simulink model "attitude_estimation_AS_V4"  (Simulink 8.9)
settings: Solver=ode45  StartTime=0.0  StopTime=400  FixedStep=T  RelTol=1e-9  EnableMultiTasking=on
values from neighbouring files (symbols this model uses):
  ARW = ARWSigma*(pi/180)/sqrt(3600)    [graficosD7.m]    (also in iattitude_estimation.m = 2.9e-06; iattitude_estimation_AS.m)
  best0 = 0    [iattitude_estimation.m]    (also in iattitude_estimation_AS.m)
  bias_cte = 4.848e-6*bias_cte    [iattitude_estimation.m]    (also in iattitude_estimation_AS.m = bias_cte*(pi/(180*3600)))
  BISigma = 0    [iattitude_estimation_AS.m]
  Misalig = [ ... (first row only)    [iattitude_estimation.m]    (also in iattitude_estimation_AS.m)
  Pest0 = zeros(6,6)    [iattitude_estimation.m]    (also in iattitude_estimation_AS.m)
  Q = 1*C_bl_GYRO_aux*Q_coefs*(C_bl_GYRO_aux')    [iattitude_estimation_AS.m]
  qest0 = qest0/sqrt(qest0'*qest0)    [iattitude_estimation.m]    (also in iattitude_estimation_AS.m)
  qreal0 = qreal0/sqrt(qreal0'*qreal0)    [iattitude_estimation.m]    (also in iattitude_estimation_AS.m)
  R = 1*(1/4)*C_bl_STR*(eye(3)*(sss^2))*(C_bl_STR')    [iattitude_estimation_AS.m]
  RRW = 8e-8*RRW    (= 0)    [iattitude_estimation.m]    (also in iattitude_estimation_AS.m)
  seta1filt = 1*ARW    (= 2.9e-06)    [iattitude_estimation.m]    (also in iattitude_estimation_AS.m = 1*ARW)
  seta2filt = 1*1e-7    (= 1e-07)    [iattitude_estimation.m]    (also in iattitude_estimation_AS.m)
  So = So/(2*3.1416)    (= 185311.942959)    [iattitude_estimation.m]    (also in iattitude_estimation_AS.m = 185312.376299)
  sstar = [sss; sss; sss]    [iattitude_estimation.m]    (also in iattitude_estimation_AS.m)
  sstarfilt = 1*sstar    [iattitude_estimation.m]    (also in iattitude_estimation_AS.m)
  T = 1    [iattitude_estimation.m]    (also in iattitude_estimation_AS.m)
  Tgyro = T/1    (= 1)    [iattitude_estimation.m]    (also in iattitude_estimation_AS.m = 0.1)
libraries: dspsrcs4 x1, simulink x1
settings Model: SuppressorTable=22 serialization::archive 11 0 6 0 0 0 11 0  Creator=INVAP  LastModifiedBy=root
settings DataIOCC: SignalLoggingName=sigsOut
settings DebuggingCC: SaveWithParameterizedLinksMsg=none  SignalResolutionControl=TryResolveAllWithWarning  MultiTaskDSMMsg=warning  MultiTaskCondExecSysMsg=none  FcnCallInpInsideContextMsg=error  StateNameClashWarn=none
settings HardwareCC: TargetUnknown=on
settings ConfigComp: CovSFcnEnable=off

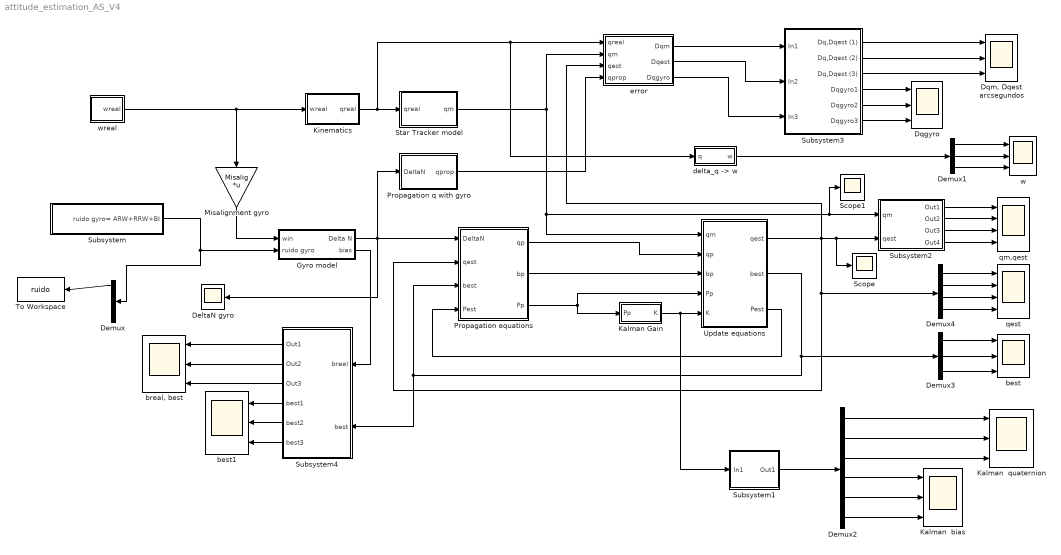
== system attitude_estimation_AS_V4 ==
  DeltaN gyro : Scope
  Demux : Demux  Outputs=3
  Demux1 : Demux  Outputs=3
  Demux2 : Demux  Outputs=6
  Demux3 : Demux  Outputs=3
  Demux4 : Demux
  Dqgyro : Scope  NumInputPorts=3
  "Dqm, Dqest arcsegundos" : Scope  NumInputPorts=3
  Gyro model : Subsystem
  Kalman Gain : Subsystem
  Kalman  bias : Scope  NumInputPorts=3
  Kalman  quaternion : Scope  NumInputPorts=3
  Kinematics : Subsystem
  Misalignment gyro : Gain  Gain=Misalig  Multiplication=Matrix(K*u) (u vector)  SaturateOnIntegerOverflow=on  OutDataTypeStr=Inherit: Same as input  ParamDataTypeStr=Inherit: Same as input
  Propagation equations : Subsystem
  Propagation q with gyro : Subsystem
  Scope : Scope
  Scope1 : Scope
  Star Tracker model : Subsystem
  Subsystem : Subsystem
  Subsystem1 : Subsystem
  Subsystem2 : Subsystem
  Subsystem3 : Subsystem
  Subsystem4 : Subsystem
  To Workspace : ToWorkspace  VariableName=ruido  SaveFormat=Timeseries  SampleTime=-1
  Update equations : Subsystem
  best : Scope  NumInputPorts=3
  best1 : Scope  NumInputPorts=3
  "breal, best" : Scope  NumInputPorts=3
  "delta_q -> w" : Subsystem
  error : Subsystem
  qest : Scope  NumInputPorts=4
  qm,qest : Scope  NumInputPorts=4
  w : Scope  NumInputPorts=3
  wreal : Subsystem
  wires:
  Kinematics/1(qreal) -> Star Tracker model/1(qreal), "delta_q -> w"/1(q), error/1(qreal)
  wreal/1(wreal) -> Kinematics/1(wreal), Misalignment gyro/1
  Star Tracker model/1(qm) -> error/2(qm), Update equations/1(qm), Scope1/1, Subsystem2/1(qm)
  Propagation equations/1(qp) -> Update equations/2(qp)
  Kalman Gain/1(K) -> Update equations/5(K), Subsystem1/1(In1)
  Update equations/3(Pest) -> Propagation equations/4(Pest)
  Update equations/1(qest) -> error/3(qest), Scope/1, Subsystem2/2(qest), Propagation equations/2(qest), Demux4/1
  Gyro model/1(Delta N) -> Propagation equations/1(DeltaN), Propagation q with gyro/1(DeltaN), DeltaN gyro/1
  Propagation q with gyro/1(qprop) -> error/4(qprop)
  Propagation equations/2(bp) -> Update equations/3(bp)
  Propagation equations/3(Pp) -> Update equations/4(Pp), Kalman Gain/1(Pp)
  Misalignment gyro/1 -> Gyro model/1(win)
  Update equations/2(best) -> Subsystem4/2(best), Propagation equations/3(best), Demux3/1
  Subsystem/1(ruido gyro= ARW+RRW+BI) -> Gyro model/2(ruido gyro), Demux/1
  Demux2/1 -> Kalman  quaternion/1
  Demux2/2 -> Kalman  quaternion/2
  Demux2/3 -> Kalman  quaternion/3
  Demux2/5 -> Kalman  bias/2
  Demux2/4 -> Kalman  bias/1
  Demux3/2 -> best/2
  Demux4/1 -> qest/1
  Demux4/2 -> qest/2
  Demux4/3 -> qest/3
  Subsystem1/1(Out1) -> Demux2/1
  Demux4/4 -> qest/4
  Subsystem2/1(Out1) -> qm,qest/1
  Subsystem2/2(Out2) -> qm,qest/2
  Subsystem2/3(Out3) -> qm,qest/3
  Subsystem2/4(Out4) -> qm,qest/4
  error/1(Dqm) -> Subsystem3/1(In1)
  error/2(Dqest) -> Subsystem3/2(In2)
  error/3(Dqgyro) -> Subsystem3/3(In3)
  Subsystem3/1(Dq,Dqest (1)) -> "Dqm, Dqest arcsegundos"/1
  Subsystem3/2(Dq,Dqest (2)) -> "Dqm, Dqest arcsegundos"/2
  Subsystem3/3(Dq,Dqest (3)) -> "Dqm, Dqest arcsegundos"/3
  Gyro model/2(bias) -> Subsystem4/1(breal)
  Subsystem3/4(Dqgyro1) -> Dqgyro/1
  Subsystem3/5(Dqgyro2) -> Dqgyro/2
  Subsystem3/6(Dqgyro3) -> Dqgyro/3
  "delta_q -> w"/1(w) -> Demux1/1
  Demux1/2 -> w/2
  Demux1/3 -> w/3
  Demux1/1 -> w/1
  Demux3/1 -> best/1
  Demux3/3 -> best/3
  Demux2/6 -> Kalman  bias/3
  Subsystem4/5(best2) -> best1/2
  Subsystem4/4(best1) -> best1/1
  Subsystem4/6(best3) -> best1/3
  Subsystem4/1(Out1) -> "breal, best"/1
  Subsystem4/2(Out2) -> "breal, best"/2
  Subsystem4/3(Out3) -> "breal, best"/3
  Demux/1 -> To Workspace/1

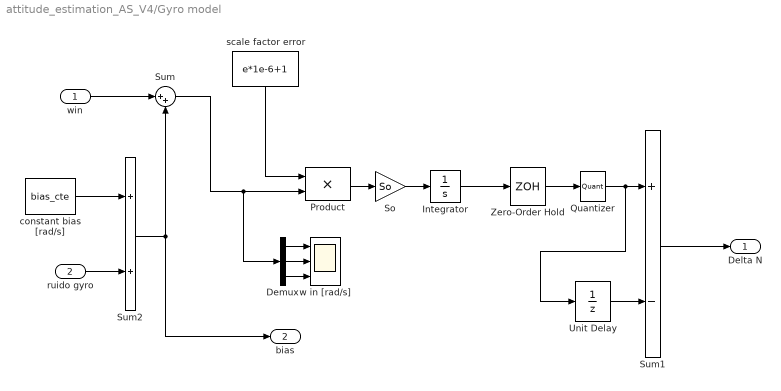
== system attitude_estimation_AS_V4/Gyro model ==
  win : Inport
  ruido gyro : Inport  Port=2
  Demux : Demux  Outputs=3
  Integrator : Integrator
  Product : Product  SaturateOnIntegerOverflow=on  OutDataTypeStr=Inherit: Same as first input
  Quantizer : Quantizer  QuantizationInterval=1
  So : Gain  Gain=So  SaturateOnIntegerOverflow=on  OutDataTypeStr=Inherit: Same as input  ParamDataTypeStr=Inherit: Same as input
  Sum : Sum  Inputs=|++  SaturateOnIntegerOverflow=on
  Sum1 : Sum  Inputs=+-  SaturateOnIntegerOverflow=on
  Sum2 : Sum  SaturateOnIntegerOverflow=on
  Unit Delay : UnitDelay  SampleTime=Tgyro
  Zero-Order Hold : ZeroOrderHold  SampleTime=Tgyro
  constant bias [rad/s] : Constant  Value=bias_cte
  scale factor error : Constant  Value=e*1e-6+1
  w in [rad/s] : Scope  NumInputPorts=3
  Delta N : Outport
  bias : Outport  Port=2
  wires:
  So/1 -> Integrator/1
  Product/1 -> So/1
  scale factor error/1 -> Product/1
  Zero-Order Hold/1 -> Quantizer/1
  Unit Delay/1 -> Sum1/2
  Integrator/1 -> Zero-Order Hold/1
  Sum1/1 -> Delta N/1
  Quantizer/1 -> Sum1/1, Unit Delay/1
  Sum2/1 -> Sum/2, bias/1
  ruido gyro/1 -> Sum2/2
  win/1 -> Sum/1
  Demux/1 -> w in [rad/s]/1
  Demux/2 -> w in [rad/s]/2
  Demux/3 -> w in [rad/s]/3
  Sum/1 -> Demux/1, Product/2
  constant bias [rad/s]/1 -> Sum2/1

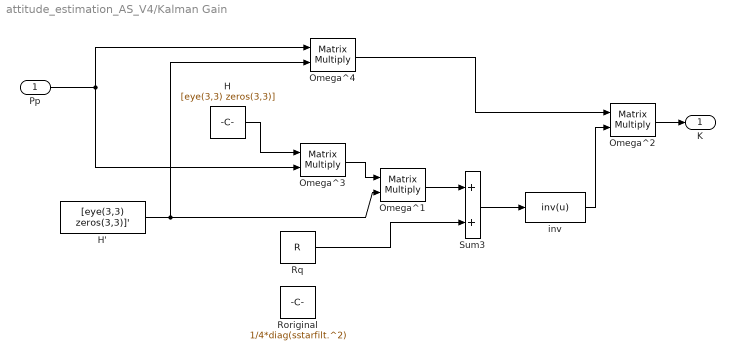
== system attitude_estimation_AS_V4/Kalman Gain ==
  Pp : Inport
  H : Constant  Value=[eye(3,3) zeros(3,3)]  VectorParams1D=off
  H' : Constant  Value=[eye(3,3) zeros(3,3)]'  VectorParams1D=off
  Omega^{1..4} (4 alike) : Product  Multiplication=Matrix(*)  SaturateOnIntegerOverflow=on  OutDataTypeStr=Inherit: Same as first input
  Roriginal : Constant  Value=1/4*diag(sstarfilt.^2)  VectorParams1D=off
  Rq : Constant  Value=R  VectorParams1D=off
  Sum3 : Sum  SaturateOnIntegerOverflow=on
  inv : MATLABFcn  MATLABFcn=inv(u)  Output1D=off
  K : Outport
  wires:
  H/1 -> Omega^3/1
  Pp/1 -> Omega^3/2, Omega^4/1
  Omega^3/1 -> Omega^1/1
  H'/1 -> Omega^1/2, Omega^4/2
  Omega^1/1 -> Sum3/1
  Omega^2/1 -> K/1
  Omega^4/1 -> Omega^2/1
  Sum3/1 -> inv/1
  inv/1 -> Omega^2/2
  Rq/1 -> Sum3/2

== system attitude_estimation_AS_V4/Kinematics ==
  wreal : Inport
  Integrator : Integrator  InitialCondition=qreal0
  MATLAB Fcn : MATLABFcn  MATLABFcn=1/2*[0 u(3) -u(2) u(1); -u(3) 0 u(1) u(2); u(2) -u(1) 0 u(3); -u(1) -u(2) -u(3) 0]  Output1D=off
  Product : Product  Multiplication=Matrix(*)  SaturateOnIntegerOverflow=on  OutDataTypeStr=Inherit: Same as first input
  qreal : Outport
  wires:
  wreal/1 -> MATLAB Fcn/1
  MATLAB Fcn/1 -> Product/1
  Product/1 -> Integrator/1
  Integrator/1 -> Product/2, qreal/1

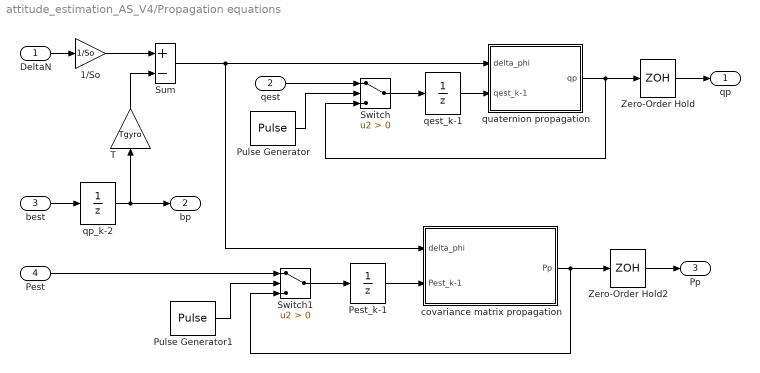
== system attitude_estimation_AS_V4/Propagation equations ==
  DeltaN : Inport
  qest : Inport  Port=2
  best : Inport  Port=3
  Pest : Inport  Port=4
  1/So : Gain  Gain=1/So  SaturateOnIntegerOverflow=on  OutDataTypeStr=Inherit: Same as input  ParamDataTypeStr=Inherit: Same as input
  Pest_k-1 : UnitDelay  InitialCondition=Pest0  SampleTime=Tgyro
  Pulse Generator : DiscretePulseGenerator  Period=T/Tgyro  SampleTime=Tgyro
  Pulse Generator1 : DiscretePulseGenerator  Period=T/Tgyro  SampleTime=Tgyro
  Sum : Sum  Inputs=+-  SaturateOnIntegerOverflow=on
  Switch : Switch  Criteria=u2 > Threshold  SaturateOnIntegerOverflow=on
  Switch1 : Switch  Criteria=u2 > Threshold  SaturateOnIntegerOverflow=on
  T : Gain  Gain=Tgyro  SaturateOnIntegerOverflow=on  OutDataTypeStr=Inherit: Same as input  ParamDataTypeStr=Inherit: Same as input
  Zero-Order Hold : ZeroOrderHold  SampleTime=T
  Zero-Order Hold2 : ZeroOrderHold  SampleTime=T
  covariance matrix propagation : Subsystem
  qest_k-1 : UnitDelay  InitialCondition=qest0  SampleTime=Tgyro
  qp_k-2 : UnitDelay  InitialCondition=best0  SampleTime=T
  quaternion propagation : Subsystem
  qp : Outport
  bp : Outport  Port=2
  Pp : Outport  Port=3
  wires:
  DeltaN/1 -> 1/So/1
  Sum/1 -> quaternion propagation/1(delta_phi), covariance matrix propagation/1(delta_phi)
  quaternion propagation/1(qp) -> Zero-Order Hold/1, Switch/3
  T/1 -> Sum/2
  1/So/1 -> Sum/1
  covariance matrix propagation/1(Pp) -> Zero-Order Hold2/1, Switch1/3
  Zero-Order Hold/1 -> qp/1
  qest/1 -> Switch/1
  Pulse Generator/1 -> Switch/2
  qest_k-1/1 -> quaternion propagation/2(qest_k-1)
  Switch/1 -> qest_k-1/1
  Pest_k-1/1 -> covariance matrix propagation/2(Pest_k-1)
  best/1 -> qp_k-2/1
  qp_k-2/1 -> bp/1, T/1
  Zero-Order Hold2/1 -> Pp/1
  Switch1/1 -> Pest_k-1/1
  Pest/1 -> Switch1/1
  Pulse Generator1/1 -> Switch1/2

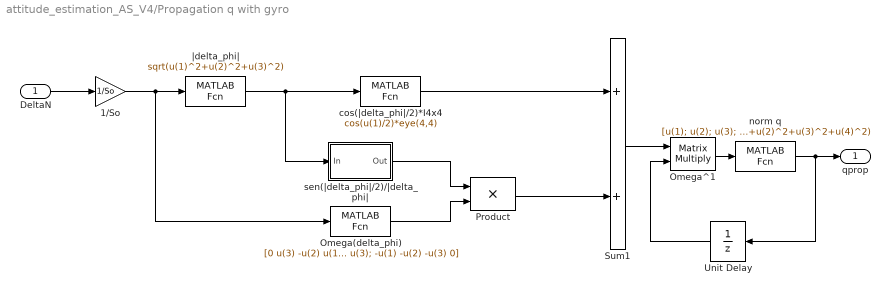
== system attitude_estimation_AS_V4/Propagation q with gyro ==
  DeltaN : Inport
  1/So : Gain  Gain=1/So  SaturateOnIntegerOverflow=on  OutDataTypeStr=Inherit: Same as input  ParamDataTypeStr=Inherit: Same as input
  Omega(delta_phi) : MATLABFcn  MATLABFcn=[0 u(3) -u(2) u(1); -u(3) 0 u(1) u(2); u(2) -u(1) 0 u(3); -u(1) -u(2) -u(3) 0]  Output1D=off
  Omega^1 : Product  Multiplication=Matrix(*)  SaturateOnIntegerOverflow=on  OutDataTypeStr=Inherit: Same as first input
  Product : Product  SaturateOnIntegerOverflow=on  OutDataTypeStr=Inherit: Same as first input
  Sum1 : Sum  SaturateOnIntegerOverflow=on
  Unit Delay : UnitDelay  InitialCondition=qreal0  SampleTime=Tgyro
  cos(|delta_phi|/2)*I4x4 : MATLABFcn  MATLABFcn=cos(u(1)/2)*eye(4,4)  Output1D=off
  norm q : MATLABFcn  MATLABFcn=[u(1); u(2); u(3); u(4)]/sqrt(u(1)^2+u(2)^2+u(3)^2+u(4)^2)  Output1D=off
  sen(|delta_phi|/2)/|delta_phi| : Subsystem
  |delta_phi| : MATLABFcn  MATLABFcn=sqrt(u(1)^2+u(2)^2+u(3)^2)  Output1D=off
  qprop : Outport
  wires:
  DeltaN/1 -> 1/So/1
  Omega^1/1 -> norm q/1
  norm q/1 -> qprop/1, Unit Delay/1
  Sum1/1 -> Omega^1/1
  Unit Delay/1 -> Omega^1/2
  |delta_phi|/1 -> cos(|delta_phi|/2)*I4x4/1, sen(|delta_phi|/2)/|delta_phi|/1(In)
  1/So/1 -> |delta_phi|/1, Omega(delta_phi)/1
  cos(|delta_phi|/2)*I4x4/1 -> Sum1/1
  Product/1 -> Sum1/2
  sen(|delta_phi|/2)/|delta_phi|/1(Out) -> Product/1
  Omega(delta_phi)/1 -> Product/2

== system attitude_estimation_AS_V4/Star Tracker model ==
  qreal : Inport
  Product : Product  Multiplication=Matrix(*)  SaturateOnIntegerOverflow=on  OutDataTypeStr=Inherit: Same as first input
  Qprim : MATLABFcn  MATLABFcn=[u(4) u(3) -u(2) u(1); -u(3) u(4) u(1) u(2); u(2) -u(1) u(4) u(3); -u(1) -u(2) -u(3) u(4)]  Output1D=off
  Zero-Order Hold : ZeroOrderHold  SampleTime=T
  "noise pitch, yaw, roll" : RandomNumber  Variance=sstar.^2  Seed=rand(3,1)*100  SampleTime=T  VectorParams1D=off
  noise_q : MATLABFcn  MATLABFcn=[1/2*u(1); 1/2*u(2); 1/2*u(3); 1]  Output1D=off
  normalition qm : MATLABFcn  MATLABFcn=[u(1); u(2); u(3); u(4)]/sqrt(u(1)^2+u(2)^2+u(3)^2+u(4)^2)  Output1D=off
  qm : Outport
  wires:
  "noise pitch, yaw, roll"/1 -> noise_q/1
  noise_q/1 -> Qprim/1
  Qprim/1 -> Product/1
  qreal/1 -> Zero-Order Hold/1
  Product/1 -> normalition qm/1
  normalition qm/1 -> qm/1
  Zero-Order Hold/1 -> Product/2

== system attitude_estimation_AS_V4/Subsystem ==
  Colored Noise : dspsrcs4/Colored Noise  Color=pink  InverseFrequencyPower=1  NumChannels=1  OutputDataType=double  SamplesPerFrame=1  SampleTime=Tgyro  RandomStream=mt19937ar with seed  Seed=67  SimulateUsing=Interpreted execution
      settings: SourceProductName=DSP System Toolbox  SourceProductBaseCode=DS
  Gain1 : Gain  Gain=ARW
  Gain2 : Gain  Gain=RRW
  Gain3 : Gain  Gain=BISigma/3600
  Integrator : Integrator
  Interpreted MATLAB Function : MATLABFcn  MATLABFcn=[u;u;u]  Output1D=off
  Random Number : RandomNumber  SampleTime=Tgyro
  Sum : Sum  Inputs=+++
  ruido gyro= ARW+RRW+BI : Outport
  wires:
  Random Number/1 -> Gain1/1, Gain2/1
  Sum/1 -> Interpreted MATLAB Function/1
  Gain1/1 -> Sum/1  "Angle random walk"
  Gain2/1 -> Integrator/1
  Interpreted MATLAB Function/1 -> ruido gyro= ARW+RRW+BI/1
  Colored Noise/1 -> Gain3/1
  Integrator/1 -> Sum/2  "Rate random walk"
  Gain3/1 -> Sum/3  "Bias instability"

== system attitude_estimation_AS_V4/Subsystem1 ==
  In1 : Inport
  Interpreted MATLAB Function : MATLABFcn  MATLABFcn=[u(1,1);u(2,2);u(3,3);u(4,1);u(5,2);u(6,3)]  Output1D=off
  Out1 : Outport
  wires:
  In1/1 -> Interpreted MATLAB Function/1
  Interpreted MATLAB Function/1 -> Out1/1

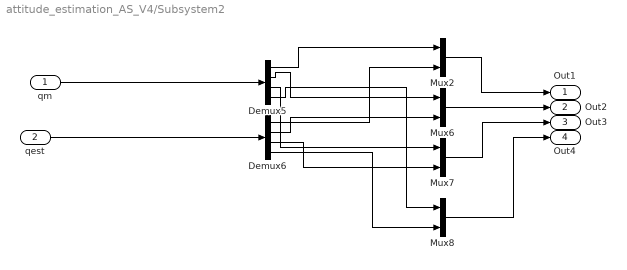
== system attitude_estimation_AS_V4/Subsystem2 ==
  qm : Inport
  qest : Inport  Port=2
  Demux5 : Demux
  Demux6 : Demux
  Mux{2,6..8} (4 alike) : Mux  Inputs=2
  Out1 : Outport
  Out2 : Outport  Port=2
  Out3 : Outport  Port=3
  Out4 : Outport  Port=4
  wires:
  qest/1 -> Demux6/1
  Demux6/3 -> Mux7/2
  Mux8/1 -> Out4/1
  Demux5/4 -> Mux8/1
  Demux5/3 -> Mux7/1
  Mux7/1 -> Out3/1
  Demux6/2 -> Mux6/2
  Demux6/4 -> Mux8/2
  qm/1 -> Demux5/1
  Demux5/1 -> Mux2/1
  Demux6/1 -> Mux2/2
  Demux5/2 -> Mux6/1
  Mux2/1 -> Out1/1
  Mux6/1 -> Out2/1

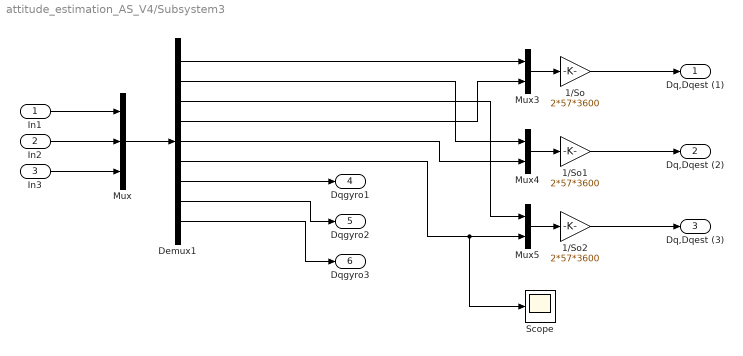
== system attitude_estimation_AS_V4/Subsystem3 ==
  In1 : Inport
  In2 : Inport  Port=2
  In3 : Inport  Port=3
  1/So : Gain  Gain=2*57*3600  SaturateOnIntegerOverflow=on  OutDataTypeStr=Inherit: Same as input  ParamDataTypeStr=Inherit: Same as input
  1/So1 : Gain  Gain=2*57*3600  SaturateOnIntegerOverflow=on  OutDataTypeStr=Inherit: Same as input  ParamDataTypeStr=Inherit: Same as input
  1/So2 : Gain  Gain=2*57*3600  SaturateOnIntegerOverflow=on  OutDataTypeStr=Inherit: Same as input  ParamDataTypeStr=Inherit: Same as input
  Demux1 : Demux  Outputs=9
  Mux : Mux  Inputs=3
  Mux3 : Mux  Inputs=2
  Mux4 : Mux  Inputs=2
  Mux5 : Mux  Inputs=2
  Scope : Scope
  Dq,Dqest (1) : Outport
  Dq,Dqest (2) : Outport  Port=2
  Dq,Dqest (3) : Outport  Port=3
  Dqgyro1 : Outport  Port=4
  Dqgyro2 : Outport  Port=5
  Dqgyro3 : Outport  Port=6
  wires:
  Demux1/8 -> Dqgyro2/1
  Demux1/2 -> Mux4/1
  1/So2/1 -> Dq,Dqest (3)/1
  Demux1/5 -> Mux4/2
  1/So1/1 -> Dq,Dqest (2)/1
  Demux1/3 -> Mux5/1
  Demux1/6 -> Scope/1, Mux5/2
  Mux5/1 -> 1/So2/1
  Demux1/4 -> Mux3/2
  Demux1/1 -> Mux3/1
  Demux1/7 -> Dqgyro1/1
  In3/1 -> Mux/3
  In2/1 -> Mux/2
  Mux/1 -> Demux1/1
  In1/1 -> Mux/1
  1/So/1 -> Dq,Dqest (1)/1
  Demux1/9 -> Dqgyro3/1
  Mux4/1 -> 1/So1/1
  Mux3/1 -> 1/So/1

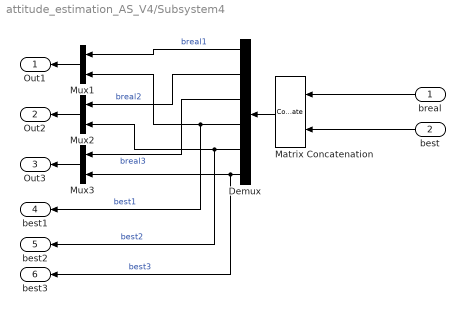
== system attitude_estimation_AS_V4/Subsystem4 ==
  breal : Inport
  best : Inport  Port=2
  Demux : Demux  Outputs=6
  Matrix Concatenation : Concatenate  Mode=Multidimensional array
  Mux1 : Mux  Inputs=2
  Mux2 : Mux  Inputs=2
  Mux3 : Mux  Inputs=2
  Out1 : Outport
  Out2 : Outport  Port=2
  Out3 : Outport  Port=3
  best1 : Outport  Port=4
  best2 : Outport  Port=5
  best3 : Outport  Port=6
  wires:
  Demux/6 -> best3/1, Mux3/2  "best3"
  Matrix Concatenation/1 -> Demux/1
  Demux/5 -> best2/1, Mux2/2  "best2"
  Mux3/1 -> Out3/1
  Mux2/1 -> Out2/1
  best/1 -> Matrix Concatenation/2
  Mux1/1 -> Out1/1
  Demux/2 -> Mux2/1  "breal2"
  Demux/4 -> best1/1, Mux1/2  "best1"
  Demux/1 -> Mux1/1  "breal1"
  breal/1 -> Matrix Concatenation/1
  Demux/3 -> Mux3/1  "breal3"

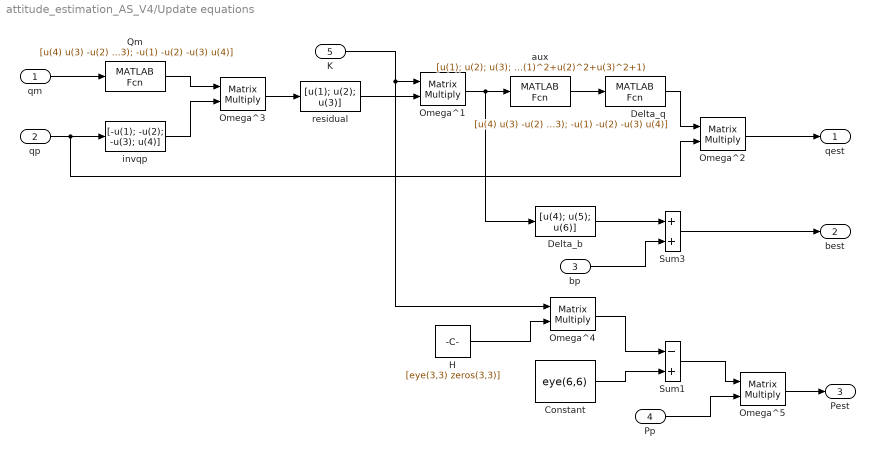
== system attitude_estimation_AS_V4/Update equations ==
  qm : Inport
  qp : Inport  Port=2
  bp : Inport  Port=3
  Pp : Inport  Port=4
  K : Inport  Port=5
  Constant : Constant  Value=eye(6,6)  VectorParams1D=off
  Delta_b : MATLABFcn  MATLABFcn=[u(4); u(5); u(6)]  Output1D=off
  Delta_q : MATLABFcn  MATLABFcn=[u(4) u(3) -u(2) u(1); -u(3) u(4) u(1) u(2); u(2) -u(1) u(4) u(3); -u(1) -u(2) -u(3) u(4)]  Output1D=off
  H : Constant  Value=[eye(3,3) zeros(3,3)]  VectorParams1D=off
  Omega^{1..5} (5 alike) : Product  Multiplication=Matrix(*)  SaturateOnIntegerOverflow=on  OutDataTypeStr=Inherit: Same as first input
  Qm : MATLABFcn  MATLABFcn=[u(4) u(3) -u(2) u(1); -u(3) u(4) u(1) u(2); u(2) -u(1) u(4) u(3); -u(1) -u(2) -u(3) u(4)]  Output1D=off
  Sum1 : Sum  Inputs=-+  SaturateOnIntegerOverflow=on
  Sum3 : Sum  SaturateOnIntegerOverflow=on
  aux : MATLABFcn  MATLABFcn=[u(1); u(2); u(3); 1]*sqrt(u(1)^2+u(2)^2+u(3)^2+1)  Output1D=off
  invqp : MATLABFcn  MATLABFcn=[-u(1); -u(2); -u(3); u(4)]  Output1D=off
  residual : MATLABFcn  MATLABFcn=[u(1); u(2); u(3)]  Output1D=off
  qest : Outport
  best : Outport  Port=2
  Pest : Outport  Port=3
  wires:
  Qm/1 -> Omega^3/1
  invqp/1 -> Omega^3/2
  Omega^3/1 -> residual/1
  qm/1 -> Qm/1
  qp/1 -> invqp/1, Omega^2/2
  residual/1 -> Omega^1/2
  K/1 -> Omega^1/1, Omega^4/1
  Omega^1/1 -> aux/1, Delta_b/1
  aux/1 -> Delta_q/1
  Delta_q/1 -> Omega^2/1
  Omega^2/1 -> qest/1
  Delta_b/1 -> Sum3/1
  Sum3/1 -> best/1
  bp/1 -> Sum3/2
  H/1 -> Omega^4/2
  Constant/1 -> Sum1/2
  Omega^4/1 -> Sum1/1
  Sum1/1 -> Omega^5/1
  Pp/1 -> Omega^5/2
  Omega^5/1 -> Pest/1

== system attitude_estimation_AS_V4/delta_q -> w ==
  q : Inport
  MATLAB Fcn : MATLABFcn  MATLABFcn=2/T*pinv([u(4) -u(3) u(2); u(3) u(4) -u(1); -u(2) u(1) u(4); -u(1) -u(2) -u(3)])  Output1D=off
  Product : Product  Multiplication=Matrix(*)  SaturateOnIntegerOverflow=on  OutDataTypeStr=Inherit: Same as first input
  Sum : Sum  Inputs=+-  SaturateOnIntegerOverflow=on
  Unit Delay : UnitDelay  SampleTime=T
  Zero-Order Hold : ZeroOrderHold  SampleTime=T
  w : Outport
  wires:
  Unit Delay/1 -> Sum/2
  Sum/1 -> Product/2
  q/1 -> Zero-Order Hold/1
  MATLAB Fcn/1 -> Product/1
  Product/1 -> w/1
  Zero-Order Hold/1 -> MATLAB Fcn/1, Sum/1, Unit Delay/1

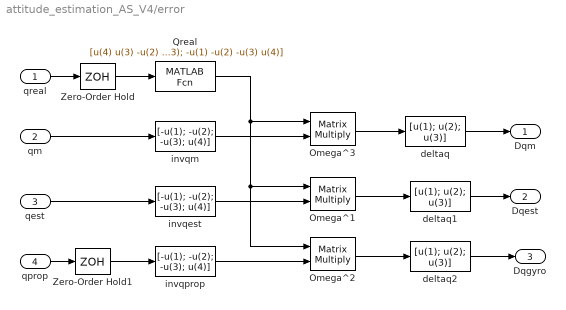
== system attitude_estimation_AS_V4/error ==
  qreal : Inport
  qm : Inport  Port=2
  qest : Inport  Port=3
  qprop : Inport  Port=4
  Omega^1 : Product  Multiplication=Matrix(*)  SaturateOnIntegerOverflow=on  OutDataTypeStr=Inherit: Same as first input
  Omega^2 : Product  Multiplication=Matrix(*)  SaturateOnIntegerOverflow=on  OutDataTypeStr=Inherit: Same as first input
  Omega^3 : Product  Multiplication=Matrix(*)  SaturateOnIntegerOverflow=on  OutDataTypeStr=Inherit: Same as first input
  Qreal : MATLABFcn  MATLABFcn=[u(4) u(3) -u(2) u(1); -u(3) u(4) u(1) u(2); u(2) -u(1) u(4) u(3); -u(1) -u(2) -u(3) u(4)]  Output1D=off
  Zero-Order Hold : ZeroOrderHold  SampleTime=T
  Zero-Order Hold1 : ZeroOrderHold  SampleTime=T
  deltaq : MATLABFcn  MATLABFcn=[u(1); u(2); u(3)]  Output1D=off
  deltaq1 : MATLABFcn  MATLABFcn=[u(1); u(2); u(3)]  Output1D=off
  deltaq2 : MATLABFcn  MATLABFcn=[u(1); u(2); u(3)]  Output1D=off
  invqest : MATLABFcn  MATLABFcn=[-u(1); -u(2); -u(3); u(4)]  Output1D=off
  invqm : MATLABFcn  MATLABFcn=[-u(1); -u(2); -u(3); u(4)]  Output1D=off
  invqprop : MATLABFcn  MATLABFcn=[-u(1); -u(2); -u(3); u(4)]  Output1D=off
  Dqm : Outport
  Dqest : Outport  Port=2
  Dqgyro : Outport  Port=3
  wires:
  Qreal/1 -> Omega^1/1, Omega^2/1, Omega^3/1
  invqm/1 -> Omega^3/2
  qreal/1 -> Zero-Order Hold/1
  Omega^3/1 -> deltaq/1
  qm/1 -> invqm/1
  qest/1 -> invqest/1
  invqest/1 -> Omega^1/2
  Omega^1/1 -> deltaq1/1
  deltaq/1 -> Dqm/1
  deltaq1/1 -> Dqest/1
  Zero-Order Hold/1 -> Qreal/1
  Omega^2/1 -> deltaq2/1
  deltaq2/1 -> Dqgyro/1
  qprop/1 -> Zero-Order Hold1/1
  invqprop/1 -> Omega^2/2
  Zero-Order Hold1/1 -> invqprop/1

== system attitude_estimation_AS_V4/wreal ==
  Manual Switch : ManualSwitch
  Ramp : simulink/Sources/Ramp  slope=[0.00001; -.000001; .0001]  start=0  X0=[0; 0; 0]  VectorParams1D=off
  wreal1 : Constant  Value=1*[0.001;-0.001;-.1]  VectorParams1D=off
  wreal : Outport
  wires:
  Manual Switch/1 -> wreal/1
  wreal1/1 -> Manual Switch/1
  Ramp/1 -> Manual Switch/2

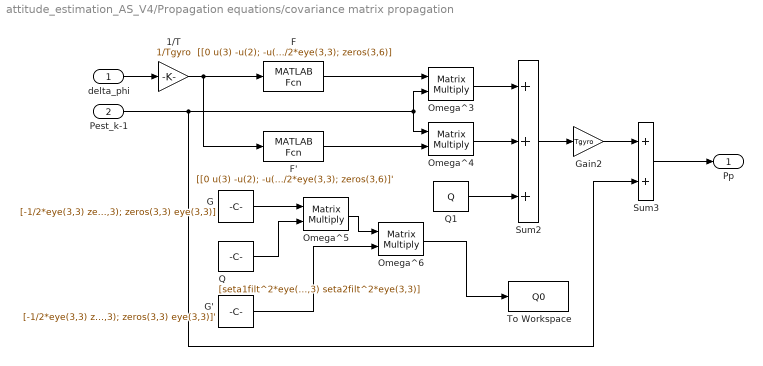
== system attitude_estimation_AS_V4/Propagation equations/covariance matrix propagation ==
  delta_phi : Inport
  Pest_k-1 : Inport  Port=2
  1/T : Gain  Gain=1/Tgyro  SaturateOnIntegerOverflow=on  OutDataTypeStr=Inherit: Same as input  ParamDataTypeStr=Inherit: Same as input
  F : MATLABFcn  MATLABFcn=[[0 u(3) -u(2); -u(3) 0 u(1); u(2) -u(1) 0] -1/2*eye(3,3); zeros(3,6)]  Output1D=off
  F' : MATLABFcn  MATLABFcn=[[0 u(3) -u(2); -u(3) 0 u(1); u(2) -u(1) 0] -1/2*eye(3,3); zeros(3,6)]'  Output1D=off
  G : Constant  Value=[-1/2*eye(3,3) zeros(3,3); zeros(3,3) eye(3,3)]  VectorParams1D=off
  G' : Constant  Value=[-1/2*eye(3,3) zeros(3,3); zeros(3,3) eye(3,3)]'  VectorParams1D=off
  Gain2 : Gain  Gain=Tgyro  SaturateOnIntegerOverflow=on  OutDataTypeStr=Inherit: Same as input  ParamDataTypeStr=Inherit: Same as input
  Omega^{3..6} (4 alike) : Product  Multiplication=Matrix(*)  SaturateOnIntegerOverflow=on  OutDataTypeStr=Inherit: Same as first input
  Q : Constant  Value=[seta1filt^2*eye(3,3) zeros(3,3); zeros(3,3) seta2filt^2*eye(3,3)]  VectorParams1D=off
  Q1 : Constant  Value=Q  VectorParams1D=off
  Sum2 : Sum  Inputs=+++  SaturateOnIntegerOverflow=on
  Sum3 : Sum  SaturateOnIntegerOverflow=on
  To Workspace : ToWorkspace  VariableName=Q0  SaveFormat=Timeseries  SampleTime=-1
  Pp : Outport
  wires:
  Sum2/1 -> Gain2/1
  Gain2/1 -> Sum3/1
  Omega^3/1 -> Sum2/1
  F/1 -> Omega^3/1
  F'/1 -> Omega^4/2
  Omega^4/1 -> Sum2/2
  G/1 -> Omega^5/1
  Q/1 -> Omega^5/2
  Omega^5/1 -> Omega^6/1
  G'/1 -> Omega^6/2
  Pest_k-1/1 -> Omega^4/1, Omega^3/2, Sum3/2
  Sum3/1 -> Pp/1
  delta_phi/1 -> 1/T/1
  1/T/1 -> F'/1, F/1
  Omega^6/1 -> To Workspace/1
  Q1/1 -> Sum2/3

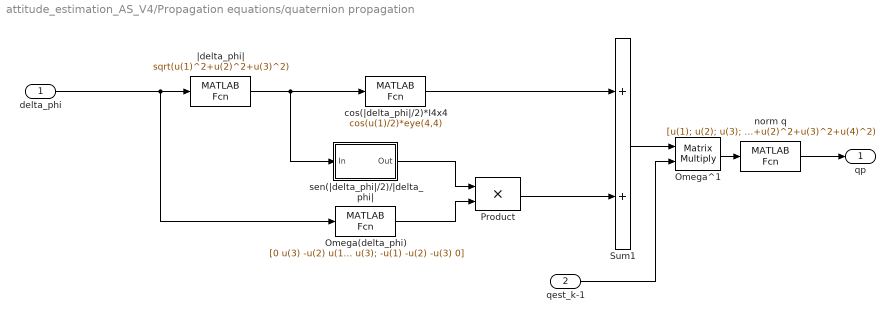
== system attitude_estimation_AS_V4/Propagation equations/quaternion propagation ==
  delta_phi : Inport
  qest_k-1 : Inport  Port=2
  Omega(delta_phi) : MATLABFcn  MATLABFcn=[0 u(3) -u(2) u(1); -u(3) 0 u(1) u(2); u(2) -u(1) 0 u(3); -u(1) -u(2) -u(3) 0]  Output1D=off
  Omega^1 : Product  Multiplication=Matrix(*)  SaturateOnIntegerOverflow=on  OutDataTypeStr=Inherit: Same as first input
  Product : Product  SaturateOnIntegerOverflow=on  OutDataTypeStr=Inherit: Same as first input
  Sum1 : Sum  SaturateOnIntegerOverflow=on
  cos(|delta_phi|/2)*I4x4 : MATLABFcn  MATLABFcn=cos(u(1)/2)*eye(4,4)  Output1D=off
  norm q : MATLABFcn  MATLABFcn=[u(1); u(2); u(3); u(4)]/sqrt(u(1)^2+u(2)^2+u(3)^2+u(4)^2)  Output1D=off
  sen(|delta_phi|/2)/|delta_phi| : Subsystem
  |delta_phi| : MATLABFcn  MATLABFcn=sqrt(u(1)^2+u(2)^2+u(3)^2)  Output1D=off
  qp : Outport
  wires:
  delta_phi/1 -> |delta_phi|/1, Omega(delta_phi)/1
  Omega^1/1 -> norm q/1
  norm q/1 -> qp/1
  Sum1/1 -> Omega^1/1
  |delta_phi|/1 -> cos(|delta_phi|/2)*I4x4/1, sen(|delta_phi|/2)/|delta_phi|/1(In)
  cos(|delta_phi|/2)*I4x4/1 -> Sum1/1
  Product/1 -> Sum1/2
  sen(|delta_phi|/2)/|delta_phi|/1(Out) -> Product/1
  Omega(delta_phi)/1 -> Product/2
  qest_k-1/1 -> Omega^1/2

== system attitude_estimation_AS_V4/Propagation q with gyro/sen(|delta_phi|/2)/|delta_phi| ==
  In : Inport
  Constant : Constant  Value=1/2
  If : If  ShowElse=off
  If Action Subsystem : Subsystem  TreatAsAtomicUnit=on
  Switch : Switch  SaturateOnIntegerOverflow=on
  Out : Outport
  wires:
  If/1 -> If Action Subsystem/Action
  If Action Subsystem/1(Out1) -> Switch/1
  Constant/1 -> Switch/3
  In/1 -> If/1, Switch/2, If Action Subsystem/1(In1)
  Switch/1 -> Out/1

== system attitude_estimation_AS_V4/Propagation equations/quaternion propagation/sen(|delta_phi|/2)/|delta_phi| ==
  In : Inport
  Constant : Constant  Value=1/2
  If : If  ShowElse=off
  If Action Subsystem : Subsystem  TreatAsAtomicUnit=on
  Switch : Switch  SaturateOnIntegerOverflow=on
  Out : Outport
  wires:
  If/1 -> If Action Subsystem/Action
  If Action Subsystem/1(Out1) -> Switch/1
  Constant/1 -> Switch/3
  In/1 -> If/1, Switch/2, If Action Subsystem/1(In1)
  Switch/1 -> Out/1

== system attitude_estimation_AS_V4/Propagation q with gyro/sen(|delta_phi|/2)/|delta_phi|/If Action Subsystem ==
  In1 : Inport
  Action Port : ActionPort  ActionType=then
  Gain : Gain  Gain=1/2  SaturateOnIntegerOverflow=on  OutDataTypeStr=Inherit: Same as input  ParamDataTypeStr=Inherit: Same as input
  Product : Product  Inputs=*/  SaturateOnIntegerOverflow=on  OutDataTypeStr=Inherit: Same as first input
  Trigonometric Function : Trigonometry
  Out1 : Outport
  wires:
  In1/1 -> Gain/1, Product/2
  Trigonometric Function/1 -> Product/1
  Product/1 -> Out1/1
  Gain/1 -> Trigonometric Function/1

== system attitude_estimation_AS_V4/Propagation equations/quaternion propagation/sen(|delta_phi|/2)/|delta_phi|/If Action Subsystem ==
  In1 : Inport
  Action Port : ActionPort  ActionType=then
  Gain : Gain  Gain=1/2  SaturateOnIntegerOverflow=on  OutDataTypeStr=Inherit: Same as input  ParamDataTypeStr=Inherit: Same as input
  Product : Product  Inputs=*/  SaturateOnIntegerOverflow=on  OutDataTypeStr=Inherit: Same as first input
  Trigonometric Function : Trigonometry
  Out1 : Outport
  wires:
  In1/1 -> Gain/1, Product/2
  Trigonometric Function/1 -> Product/1
  Product/1 -> Out1/1
  Gain/1 -> Trigonometric Function/1
